simulink model "CraneModel"  (R2021b)
settings: Solver=VariableStepAuto  StartTime=0.0  StopTime=10  MaxStep=0.00005  RelTol=1e-3
values from neighbouring files (symbols this model uses):
  B_l = 20    [TestYController.m]
  B_x = 10    [TestYController.m]
  cFrictionL = 90    [TestYController.m]
  cFrictionX = 15    [TestYController.m]
  finalStepValue = 0    [TestYController.m]
  g = 9.82    [TestYController.m]
  GravityComp = -2.73    [TestYController.m]
  I_LCurrent = 0.25    [TestYController.m]
  I_LEnd = 3    [TestYController.m]
  I_LStart = 1    [TestYController.m]
  I_xCurrent = 0    [TestYController.m]
  I_xEnd = 3    [TestYController.m]
  I_xStart = 1    [TestYController.m]
  InitStepValue = 1.25    [TestYController.m]
  InitWireLength = 1.25    [TestYController.m]
  J_l = 0.2    [TestYController.m]
  J_x = 0.2    [TestYController.m]
  k_el = 0.71    [TestYController.m]
  k_ex = 0.609    [TestYController.m]
  m_l = 0.95    [TestYController.m]
  m_t = 0.729    [TestYController.m]
  r_l = 0.05    [TestYController.m]
  r_x = 0.075    [TestYController.m]
  sFrictionL = 50    [TestYController.m]
  sFrictionX = 20    [TestYController.m]
libraries: simulink x13, slpidlib x1
settings Model: Creator=laula  LastModifiedBy=Jakob Gammelgaard

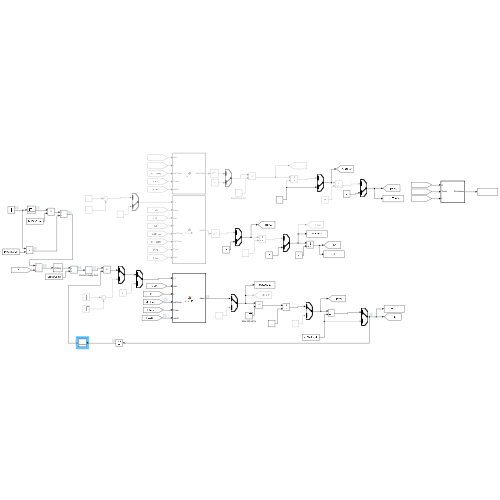
[thumbnail: Simulink's stored preview of the top-level diagram]
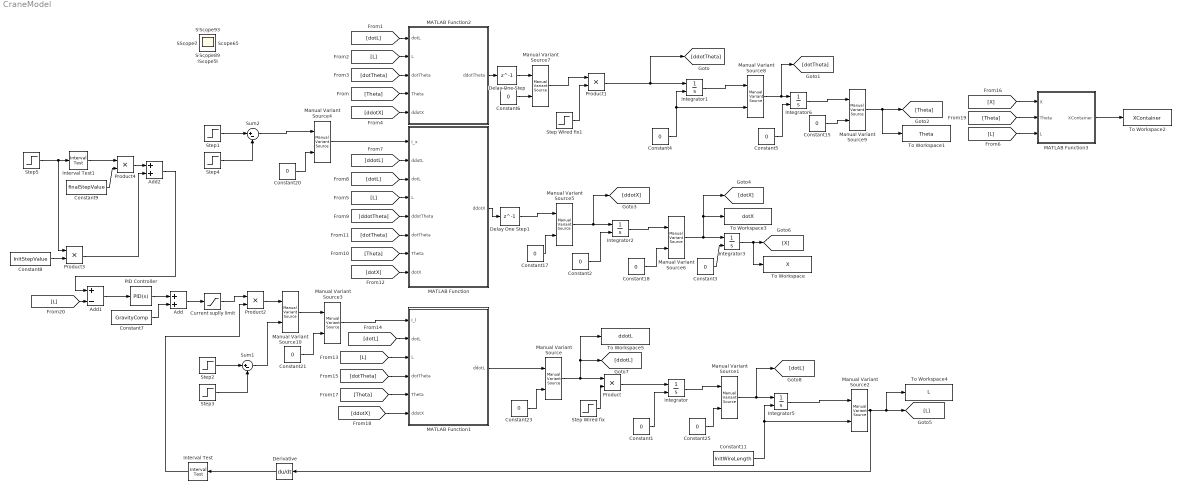
== system CraneModel ==
  Add : Sum
  Add1 : Sum  Inputs=+-
  Add2 : Sum
  Constant{1..6,15,17..18,20..21,23,25} (13 alike) : Constant  Value=0
  Constant11 : Constant  Value=InitWireLength
  Constant7 : Constant  Value=GravityComp
  Constant8 : Constant  Value=InitStepValue
  Constant9 : Constant  Value=finalStepValue
  Current suplly limit : Saturate  UpperLimit=10  LowerLimit=-10
  Delay One Step : Delay  DelayLength=1
  Delay One Step1 : Delay  DelayLength=1
  Derivative : Derivative
  Integrator{,1..3,5..6} (6 alike) : Integrator  InitialConditionSource=external
  Interval Test : simulink/Logic and Bit Operations/Interval Test  IntervalClosedRight=on  uplimit=0.55  IntervalClosedLeft=on  lowlimit=-0.55  OutDataTypeStr=boolean
  Interval Test1 : simulink/Logic and Bit Operations/Interval Test  IntervalClosedRight=on  uplimit=0.1  IntervalClosedLeft=on  lowlimit=-0.1  OutDataTypeStr=boolean
  MATLAB Function : MATLAB Function  TreatAsAtomicUnit=on
  MATLAB Function1 : MATLAB Function  TreatAsAtomicUnit=on
  MATLAB Function2 : MATLAB Function  TreatAsAtomicUnit=on
  MATLAB Function3 : MATLAB Function  TreatAsAtomicUnit=on
  Manual Variant Source{,1..3,10} (5 alike) : simulink/Signal Routing/Manual Variant Source  NumChoices=2  LabelModeActiveChoice=V_1
  Manual Variant Source{4..9} (6 alike) : simulink/Signal Routing/Manual Variant Source  NumChoices=2  LabelModeActiveChoice=V_2
  PID Controller : slpidlib/PID Controller  Controller=PID  Form=Parallel  TimeDomain=Continuous-time  UseExternalTs=off  SampleTime=-1  IntegratorMethod=Forward Euler  FilterMethod=Forward Euler  ControllerParametersSource=internal  P=150  I=0  D=75  UseFilter=on  N=100  TunerSelectOption=Transfer Function Based (PID Tuner App)  InitialConditionSource=internal  InitialConditionForIntegrator=0  InitialConditionForFilter=0  DifferentiatorICPrevScaledInput=0  ExternalReset=none  TrackingMode=off  Kt=1  LimitOutput=off  SatLimitsSource=internal  UpperSaturationLimit=inf  LowerSaturationLimit=-inf  LinearizeAsGain=on  AntiWindupMode=none  Kb=1  POutMin=[]  POutMax=[]  IOutMin=[]  IOutMax=[]  DOutMin=[]  DOutMax=[]  NOutMin=[]  NOutMax=[]  SumOutMin=[]  SumOutMax=[]  SaturationOutMin=[]  SaturationOutMax=[]  PParamMin=[]  PParamMax=[]  IParamMin=[]  IParamMax=[]  DParamMin=[]  DParamMax=[]  NParamMin=[]  NParamMax=[]  KbParamMin=[]  KbParamMax=[]  KtParamMin=[]  KtParamMax=[]  KbOutMin=[]  KbOutMax=[]  KtOutMin=[]  KtOutMax=[]  IntegratorOutMin=[]  IntegratorOutMax=[]  FilterOutMin=[]  FilterOutMax=[]  SumI1OutMin=[]  SumI1OutMax=[]  SumI2OutMin=[]  SumI2OutMax=[]  SumI3OutMin=[]  SumI3OutMax=[]  SumI4OutMin=[]  SumI4OutMax=[]  SumDOutMin=[]  SumDOutMax=[]  DifferentiatorOutMin=[]  DifferentiatorOutMax=[]  FilterDiffOutCoefMin=[]  FilterDiffOutCoefMax=[]  ReciprocalOutMin=[]  ReciprocalOutMax=[]  SumDenOutMin=[]  SumDenOutMax=[]  SumNumOutMin=[]  SumNumOutMax=[]  DivideOutMin=[]  DivideOutMax=[]  UdiffTsProdOutMin=[]  UdiffTsProdOutMax=[]  NTsProdOutMin=[]  NTsProdOutMax=[]  UintegralTsProdOutMin=[]  UintegralTsProdOutMax=[]  UngainTsProdOutMin=[]  UngainTsProdOutMax=[]  IntegratorContinuousStateAttributes=''  IntegratorStateMustResolveToSignalObject=off  IntegratorRTWStateStorageClass=Auto  FilterContinuousStateAttributes=''  FilterStateMustResolveToSignalObject=off  FilterRTWStateStorageClass=Auto  ParallelPVariant=InternalParameters  IdealPVariant=Disabled  IVariant=InternalParameters  DVariant=InternalParameters  IntegratorVariant=Continuous  SatVariant=Disabled  AWVariant=Passthrough  PCopyVariant=Disabled  TRVariant=Disabled  FdbkBlocksVariant=Forward  IdealPFdbkVariant=Disabled  SatFdbkVariant=Disabled  DerivativeFilterVariant=ContFilter  NVariant=InternalParameters  NCopyVariant=Disabled  FilterICVariant=InternalICsFilter  IntegratorICVariant=InternalICs  ExternalResetVariant=Disabled  TRSumVariant=Passthrough  SumFdbkVariant=Disabled  SumVariant=Sum_PID  TsampFilterVariant=InternalTs  TsampNgainVariant=Passthrough  TsampIntegralVariant=Passthrough  ExternalSaturationOutDataTypeStr=Inherit: Same as second input
  Product{,1..4} (5 alike) : Product
  Step Wired fix : Step  Time=0.0001  SampleTime=0
  Step Wired fix1 : Step  Time=0.001  SampleTime=0
  Step1 : Step  Time=I_xStart  After=I_xCurrent  SampleTime=0
  Step2 : Step  Time=I_LStart  After=I_LCurrent  SampleTime=0
  Step3 : Step  Time=I_LEnd  After=I_LCurrent  SampleTime=0
  Step4 : Step  Time=I_xEnd  After=I_xCurrent  SampleTime=0
  Step5 : Step  Before=1  After=0  SampleTime=0
  Sum1 : Sum  Inputs=|+-
  Sum2 : Sum  Inputs=|+-
  To Workspace : ToWorkspace  VariableName=X  SampleTime=-1
  To Workspace1 : ToWorkspace  VariableName=Theta  SampleTime=-1
  To Workspace2 : ToWorkspace  VariableName=XContainer  SampleTime=-1
  To Workspace3 : ToWorkspace  VariableName=dotX  SampleTime=-1
  To Workspace4 : ToWorkspace  VariableName=L  SampleTime=-1
  To Workspace5 : ToWorkspace  VariableName=ddotL  SampleTime=-1
  Scope{,1..26} (27 alike) : Scope
  wires:
  [dotL] -> MATLAB Function2/1(dotL)
  [L] -> MATLAB Function2/2(L)
  [dotTheta] -> MATLAB Function2/3(dotTheta)
  [Theta] -> MATLAB Function2/4(Theta)
  [ddotX] -> MATLAB Function2/5(ddotX)
  [ddotL] -> MATLAB Function/2(ddotL)
  [dotL] -> MATLAB Function/3(dotL)
  [L] -> MATLAB Function/4(L)
  [ddotTheta] -> MATLAB Function/5(ddotTheta)
  [dotTheta] -> MATLAB Function/6(dotTheta)
  [Theta] -> MATLAB Function/7(Theta)
  [ddotX] -> MATLAB Function1/6(ddotX)
  [Theta] -> MATLAB Function1/5(Theta)
  [dotTheta] -> MATLAB Function1/4(dotTheta)
  [L] -> MATLAB Function1/3(L)
  [dotL] -> MATLAB Function1/2(dotL)
  Step4/1 -> Sum2/2
  Step1/1 -> Sum2/1
  MATLAB Function/1(ddotX) -> Delay One Step1/1
  Constant3/1 -> Integrator3/2
  Constant1/1 -> Integrator/2
  Constant4/1 -> Manual Variant Source8/2, Integrator1/2
  MATLAB Function2/1(ddotTheta) -> Delay One Step/1
  [dotX] -> MATLAB Function/8(dotX)
  Integrator3/1 -> To Workspace/1, [X]
  [L] -> MATLAB Function3/3(L)
  [X] -> MATLAB Function3/1(X)
  [Theta] -> MATLAB Function3/2(Theta)
  MATLAB Function3/1(XContainer) -> To Workspace2/1
  Step2/1 -> Sum1/1
  Step3/1 -> Sum1/2
  Constant11/1 -> Manual Variant Source2/2, Integrator5/2
  Step Wired fix/1 -> Product/2
  Manual Variant Source8/1 -> Integrator6/1, [dotTheta]
  Constant5/1 -> Integrator6/2
  Manual Variant Source5/1 -> [ddotX], Integrator2/1
  Constant2/1 -> Integrator2/2
  Manual Variant Source6/1 -> [dotX], To Workspace3/1, Integrator3/1
  Manual Variant Source4/1 -> MATLAB Function/1(I_x)
  Manual Variant Source3/1 -> MATLAB Function1/1(I_l)
  Manual Variant Source/1 -> To Workspace5/1, [ddotL], Product/1
  Product/1 -> Integrator/1
  Manual Variant Source1/1 -> [dotL], Integrator5/1
  MATLAB Function1/1(ddotL) -> Manual Variant Source/1
  Constant23/1 -> Manual Variant Source/2
  Constant25/1 -> Manual Variant Source1/2
  Integrator/1 -> Manual Variant Source1/1
  Integrator5/1 -> Manual Variant Source2/1
  Constant21/1 -> Manual Variant Source3/2
  Sum2/1 -> Manual Variant Source4/1
  Constant20/1 -> Manual Variant Source4/2
  Delay One Step1/1 -> Manual Variant Source5/1
  Constant17/1 -> Manual Variant Source5/2
  Constant18/1 -> Manual Variant Source6/2
  Integrator2/1 -> Manual Variant Source6/1
  Delay One Step/1 -> Manual Variant Source7/1
  Constant6/1 -> Manual Variant Source7/2
  Integrator1/1 -> Manual Variant Source8/1
  Manual Variant Source9/1 -> To Workspace1/1, [Theta]
  Integrator6/1 -> Manual Variant Source9/1
  Constant15/1 -> Manual Variant Source9/2
  Step Wired fix1/1 -> Product1/2
  Manual Variant Source7/1 -> Product1/1
  Product1/1 -> [ddotTheta], Integrator1/1
  Manual Variant Source10/1 -> Manual Variant Source3/1
  Sum1/1 -> Manual Variant Source10/2
  Add/1 -> Current suplly limit/1
  PID Controller/1 -> Add/1
  Add1/1 -> PID Controller/1
  [L] -> Add1/2
  Manual Variant Source2/1 -> Derivative/1, To Workspace4/1, [L]
  Product2/1 -> Manual Variant Source10/1
  Current suplly limit/1 -> Product2/1
  Derivative/1 -> Interval Test/1
  Interval Test/1 -> Product2/2
  Constant7/1 -> Add/2
  Constant8/1 -> Product3/2
  Step5/1 -> Interval Test1/1, Product3/1
  Interval Test1/1 -> Product4/1
  Constant9/1 -> Product4/2
  Product4/1 -> Add2/1
  Product3/1 -> Add2/2
  Add2/1 -> Add1/1

== matlab function CraneModel/MATLAB Function1 ==
  data: I_l input; ddotL output; dotL input; L input; dotTheta input; Theta input; ddotX input; k_el parameter; r_l parameter; J_l parameter; m_l parameter; g parameter; B_l parameter; cFrictionL parameter; sFrictionL parameter
function ddotL = fcn5_13(I_l, dotL, L, dotTheta, Theta, ddotX, k_el, r_l, J_l, m_l, g, B_l,cFrictionL, sFrictionL)

if(norm(dotL)<0.05)
    friction = sFrictionL*sign(dotL);
else
    friction = B_l*dotL+cFrictionL*sign(dotL);
end


temp = -m_l*ddotX*sin(Theta);

temp = temp + m_l*L*dotTheta^2;

temp = temp; + m_l*g*cos(Theta);

temp = temp -friction;

temp = temp + 2*k_el*I_l/r_l;

ddotL=temp/(m_l+4*J_l/r_l^2);

== matlab function CraneModel/MATLAB Function ==
  data: I_x input; ddotX output; ddotL input; dotL input; L input; ddotTheta input; dotTheta input; Theta input; dotX input; J_x parameter; r_x parameter double; k_ex parameter; m_t parameter; m_l parameter; B_x parameter; sFrictionX parameter; cFrictionX parameter
function ddotX = fcn5_10(I_x, ddotL, dotL, L, ddotTheta, dotTheta, Theta, dotX, J_x, r_x, k_ex, m_t, m_l, B_x,sFrictionX, cFrictionX)

if(norm(dotX)<0.05)
    friction = sFrictionX*sign(dotX);
else
    friction = B_x*dotX+cFrictionX*sign(dotX);
end


temp = I_x*k_ex/r_x;

temp = temp  - m_l*ddotL*sin(Theta);

temp= temp -2*m_l*dotL*dotTheta*cos(Theta);

temp = temp - m_l*L*ddotTheta*cos(Theta);

temp = temp + m_l*L*(dotTheta^2)*sin(Theta);

temp = temp - friction;

temp = temp/(m_t+m_l+J_x/(r_x^2));

ddotX = temp;

== matlab function CraneModel/MATLAB Function2 ==
  data: ddotTheta output; dotL input; L input; dotTheta input; Theta input; ddotX input; g parameter
function ddotTheta = fcn5_7(dotL, L, dotTheta, Theta,ddotX,g)

temp = -2*dotL*dotTheta;

temp = temp - ddotX*cos(Theta);

temp = temp - g*sin(Theta);

temp = temp/L;

ddotTheta = temp;

== matlab function CraneModel/MATLAB Function3 ==
  data: X input; XContainer output; Theta input; L input
function XContainer = fcn(X,Theta,L)

XContainer = X + sin(Theta)*L;
